simulink model "Kursovoy"  (Simulink 8.5)
settings: Solver=ode45  StartTime=0.0  StopTime=0.2  MaxStep=10e-6  RelTol=1e-3
values from neighbouring files (symbols this model uses):
  h_r = 0.9    [Drive1.m]    (also in Drive2.m; Drive3.m)
  i_r = 286.69    [Drive1.m]    (also in Drive2.m = 841.031; Drive3.m = 768.175)
  k_m = 0.704    [Drive1.m]    (also in Drive2.m; Drive3.m = 0.764)
  k_p = 2.57E+4    (= 25700)    [Drive1.m]    (also in Drive2.m = 2577; Drive3.m = 2110)
  k_s = 2.242E+10    (= 22420000000)    [Drive1.m]    (also in Drive2.m = 3676000000; Drive3.m = 3169000000)
  k_t = 1.787    [Drive1.m]    (also in Drive2.m; Drive3.m = 7.192)
  Mdist_max = 1.294E+3    (= 1294)    [Drive1.m]    (also in Drive2.m = 14610; Drive3.m = 5081)
  Q_s = 1.049    [Drive1.m]    (also in Drive2.m = 0.376; Drive3.m = 0.265)
  T = 3.333E-6    (= 3.333e-06)    [Drive1.m]    (also in Drive2.m; Drive3.m)
  T1 = 0.23    [Drive1.m]    (also in Drive2.m = 0.485; Drive3.m = 0.391)
  T2 = 0.039    [Drive1.m]    (also in Drive2.m = 0.076; Drive3.m = 0.063)
  T5 = 5.559E-6    (= 5.559e-06)    [Drive1.m]    (also in Drive2.m = 1.08e-05; Drive3.m = 9.042e-06)
  Tau = 6.063E-4    (= 0.0006063)    [Drive1.m]    (also in Drive2.m = 0.001169; Drive3.m = 0.0009746)
  Te = 5.977E-3    (= 0.005977)    [Drive1.m]    (also in Drive2.m; Drive3.m = 0.003956)
  Tm = 0.093    [Drive1.m]    (also in Drive2.m = 0.035; Drive3.m = 0.033)
  w_max = 1.096    [Drive1.m]    (also in Drive2.m = 0.374; Drive3.m = 0.409)
  w_s = 1.044    [Drive1.m]    (also in Drive2.m = 0.993; Drive3.m = 1.543)
libraries: simulink x1
settings Model: Creator=divaise  LastModifiedBy=Admin
settings DebuggingCC: SolverPrmCheckMsg=warning  FcnCallInpInsideContextMsg=UseLocalSettings

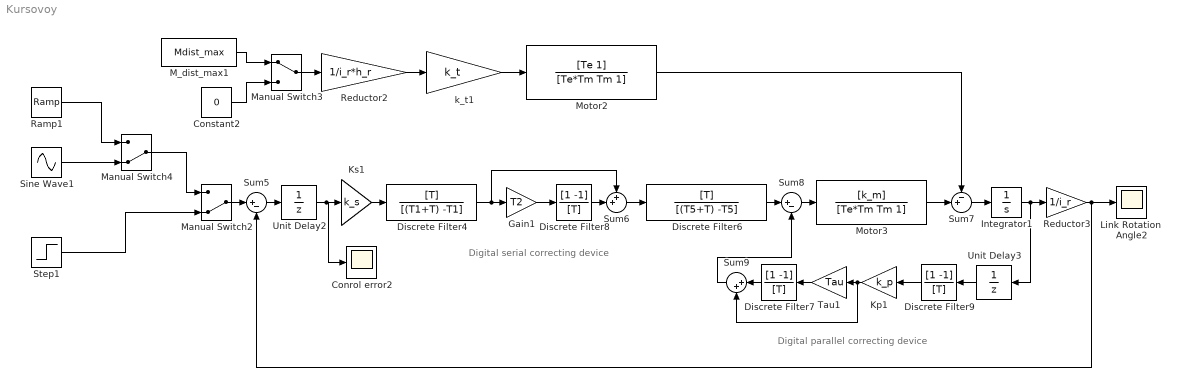
== system Kursovoy ==
  note: Digital serial correcting device
  note: Digital parallel correcting device
  Conrol error2 : Scope
      settings: TimeRange=2  YMin=0  YMax=0.0012
  Constant2 : Constant  Value=0
  Discrete Filter4 : DiscreteFilter  Numerator=[T]  Denominator=[(T1+T) -T1]  SampleTime=T
  Discrete Filter6 : DiscreteFilter  Numerator=[T]  Denominator=[(T5+T) -T5]  SampleTime=T
  Discrete Filter7 : DiscreteFilter  Numerator=[1 -1]  Denominator=[T]  SampleTime=T
  Discrete Filter8 : DiscreteFilter  Numerator=[1 -1]  Denominator=[T]  SampleTime=T
  Discrete Filter9 : DiscreteFilter  Numerator=[1 -1]  Denominator=[T]  SampleTime=T
  Gain1 : Gain  Gain=T2
  Integrator1 : Integrator
  Kp1 : Gain  Gain=k_p
  Ks1 : Gain  Gain=k_s
  Link Rotation  Angle2 : Scope
      settings: TimeRange=0.1500000000000004  YMin=-2.25e+183  YMax=5e+182
  M_dist_max1 : Constant  Value=Mdist_max
  Manual Switch2 : ManualSwitch  CurrentSetting=0
  Manual Switch3 : ManualSwitch
  Manual Switch4 : ManualSwitch  CurrentSetting=0
  Motor2 : TransferFcn  Numerator=[Te 1]  Denominator=[Te*Tm Tm 1]
  Motor3 : TransferFcn  Numerator=[k_m]  Denominator=[Te*Tm Tm 1]
  Ramp1 : simulink/Sources/Ramp  slope=w_max  start=0  X0=0
  Reductor2 : Gain  Gain=1/i_r*h_r
  Reductor3 : Gain  Gain=1/i_r
  Sine Wave1 : Sin  Amplitude=Q_s  Frequency=w_s  SampleTime=0
  Step1 : Step  Time=0  SampleTime=0
  Sum5 : Sum  Inputs=|+-
  Sum6 : Sum  Inputs=++|
  Sum7 : Sum  Inputs=-+|
  Sum8 : Sum  Inputs=|+-
  Sum9 : Sum  Inputs=|++
  Tau1 : Gain  Gain=Tau
  Unit Delay2 : UnitDelay  SampleTime=T
  Unit Delay3 : UnitDelay  SampleTime=T
  k_t1 : Gain  Gain=k_t
  wires:
  Ramp1/1 -> Manual Switch4/1
  Sine Wave1/1 -> Manual Switch4/2
  Step1/1 -> Manual Switch2/2
  Manual Switch2/1 -> Sum5/1
  Reductor2/1 -> k_t1/1
  k_t1/1 -> Motor2/1
  Sum6/1 -> Discrete Filter6/1
  Motor3/1 -> Sum7/2
  Sum7/1 -> Integrator1/1
  Integrator1/1 -> Unit Delay3/1, Reductor3/1
  Reductor3/1 -> Link Rotation  Angle2/1, Sum5/2
  Kp1/1 -> Sum9/2, Tau1/1
  Motor2/1 -> Sum7/1
  Unit Delay2/1 -> Conrol error2/1, Ks1/1
  Ks1/1 -> Discrete Filter4/1
  Discrete Filter4/1 -> Sum6/1, Gain1/1
  Discrete Filter6/1 -> Sum8/1
  Sum8/1 -> Motor3/1
  Sum9/1 -> Sum8/2
  Discrete Filter9/1 -> Kp1/1
  Tau1/1 -> Discrete Filter7/1
  Discrete Filter7/1 -> Sum9/1
  Discrete Filter8/1 -> Sum6/2
  Gain1/1 -> Discrete Filter8/1
  Sum5/1 -> Unit Delay2/1
  Unit Delay3/1 -> Discrete Filter9/1
  Manual Switch4/1 -> Manual Switch2/1
  Manual Switch3/1 -> Reductor2/1
  M_dist_max1/1 -> Manual Switch3/1
  Constant2/1 -> Manual Switch3/2
